simulink model "Tire_Force_Observer_Test"  (R2018b)
settings: Solver=VariableStepAuto  StartTime=0.0  StopTime=10  RelTol=1e-3  EnableMultiTasking=on
undefined symbols (not defined in the file or in its folder): A_s, B_s, C_s, Jw, K_s, r, sigbuilder_block, tyre_radius
libraries: simulink x1
settings Model: PauseTimes=1  Creator=univ4123  LastModifiedBy=univ4123
settings OptimizationCC: LifeSpan=inf
settings DebuggingCC: SFUnexpectedBacktrackingDiag=warning  SFNoUnconditionalDefaultTransitionDiag=warning
settings SFSimCC: SimUseLocalCustomCode=off
settings RTWCC: RTWUseLocalCustomCode=off
settings CodeAppCC: StateflowObjectComments=on
settings GRTTargetCC: TargetLangStandard=C89/C90 (ANSI)  GeneratePreprocessorConditionals=Disable all
settings ConfigComp: CovMetricSettings=dw  CovHtmlReporting=on  CovSaveCumulativeToWorkspaceVar=on  CovSaveSingleToWorkspaceVar=on  CovExternalEMLEnable=off

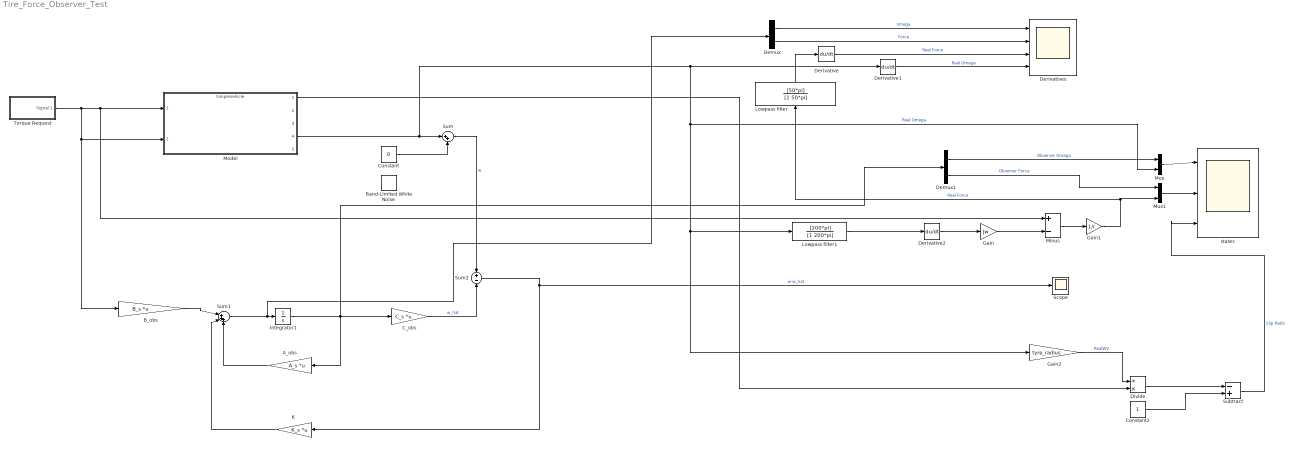
== system Tire_Force_Observer_Test ==
  A_obs : Gain  Gain=A_s  Multiplication=Matrix(K*u) (u vector)
  B_obs : Gain  Gain=B_s  Multiplication=Matrix(K*u) (u vector)
  Band-Limited White Noise : simulink/Sources/Band-Limited White Noise  Cov=[0.00001]  Ts=0.1  seed=[23341]
  C_obs : Gain  Gain=C_s  Multiplication=Matrix(K*u) (u vector)
  Constant : Constant  Value=0
  Constant2 : Constant
  Demux : Demux  Outputs=2
  Demux1 : Demux  Outputs=2
  Derivative : Derivative
  Derivative1 : Derivative
  Derivative2 : Derivative
  "Derivatives " : Scope  NumInputPorts=4
  Divide : Product  Inputs=/*
  Gain : Gain  Gain=Jw
  Gain1 : Gain  Gain=1/r
  Gain2 : Gain  Gain=tyre_radius
  Integrator1 : Integrator
  K : Gain  Gain=K_s  Multiplication=Matrix(K*u)
  Lowpass filter : TransferFcn  Numerator=[50*pi]  Denominator=[1 50*pi]
  Lowpass filter1 : TransferFcn  Numerator=[200*pi]  Denominator=[1 200*pi]
  Minus : Sum  Inputs=+-
  Model : ModelReference  ModelNameDialog=SimpleVehicle.slx  SimulationMode=Normal  ModelReferenceVersion=1.9
  Mux : Mux  Inputs=2
  Mux1 : Mux  Inputs=2
  Scope : Scope
  Subtract : Sum  Inputs=-+
  Sum : Sum  Inputs=|++
  Sum1 : Sum  Inputs=|+++
  Sum2 : Sum  Inputs=+|-
  Torque Request : Subsystem  Tag=STV Subsys  LoadFcn=sigbuilder_block('load');  StartFcn=sigbuilder_block('start');  StopFcn=sigbuilder_block('stop');  ClipboardFcn=sigbuilder_block('clipboard');  mask(Sigbuilder block){tuvar=[0:10]}
      mask help: Simulink:masks:SigbuilderBlock_MD
      mask init:
      | if ~strcmp(get_param(bdroot(gcbh),'SimulationStatus'),'stopped') tuvar = sigbuilder_block('maskInit'); end
      settings: CopyFcn=sigbuilder_block('copy');  DeleteFcn=sigbuilder_block('delete');  ModelCloseFcn=sigbuilder_block('modelClose');  PreSaveFcn=sigbuilder_block('preSave');  PauseFcn=sigbuilder_block('pause');  ContinueFcn=sigbuilder_block('continue');  NameChangeFcn=sigbuilder_block('namechange');  OpenFcn=sigbuilder_block('open',[437.6 153.75 550.4 359.25 ]);  CloseFcn=sigbuilder_block('close');
      mask Display: plot(0, 0, 100, 100,[2, 2, 32, 32, 2], [68, 8, 8, 68, 68],[32, 2], [38, 38], [32, 19, 2],[53, 60, 44], [32, 17, 17, 2],[16, 16, 31, 31]);txt = getActiveGroup(gcbh);text(2, 100, txt,'verticalAlignment', 'top');
  states : Scope  NumInputPorts=3
  wires:
  Sum1/1 -> Demux/1, Integrator1/1
  Demux1/1 -> Mux/1  "Observer Omega"
  Model/4 -> Gain2/1, Lowpass filter1/1, Mux/2, Derivative1/1, Sum/1  "Real Omega"
  Derivative/1 -> "Derivatives "/3  "Real Force"
  Sum/1 -> Sum2/1  "w"
  Integrator1/1 -> Demux1/1, A_obs/1, C_obs/1
  Constant/1 -> Sum/2
  B_obs/1 -> Sum1/1
  Demux1/2 -> Mux1/1  "Observer Force"
  Demux/2 -> "Derivatives "/2  "Force"
  A_obs/1 -> Sum1/3
  Demux/1 -> "Derivatives "/1  "omega"
  Torque Request/1(Signal 1) -> Model/1, Minus/1, Model/2, B_obs/1
  K/1 -> Sum1/2
  C_obs/1 -> Sum2/2  "w_hat"
  Sum2/1 -> Scope/1, K/1  "w-w_hat"
  Derivative1/1 -> "Derivatives "/4  "Real Omega"
  Derivative2/1 -> Gain/1
  Gain/1 -> Minus/2
  Minus/1 -> Gain1/1
  Gain1/1 -> Lowpass filter/1, Mux1/2  "Real Force"
  Gain2/1 -> Divide/1  "RealWV"
  Divide/1 -> Subtract/1
  Subtract/1 -> states/3  "Slip Ratio"
  Model/1 -> Divide/2
  Constant2/1 -> Subtract/2
  Mux/1 -> states/1
  Mux1/1 -> states/2
  Lowpass filter/1 -> Derivative/1
  Lowpass filter1/1 -> Derivative2/1

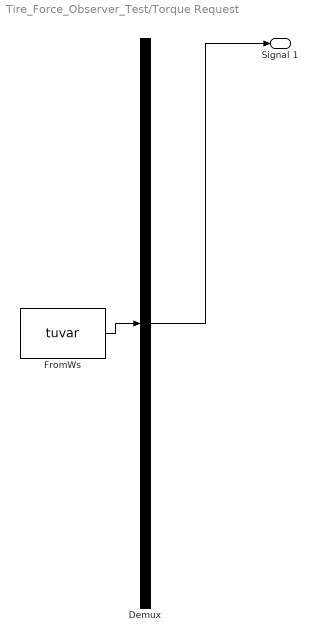
== system Tire_Force_Observer_Test/Torque Request ==
  Demux : Demux  Tag=STV Demux  Outputs=1
  FromWs : FromWorkspace  Tag=STV FromWs  VariableName=tuvar  SampleTime=0
      SigBuilderData=|
      | common.afterFinalStr = 'Extrapolate'
      | common.sampleTime = 0
      | dataSet.timeRange = [0 10]
      | dataSet.name = 'Group 1'
      | sbobj.Groups.Name = 'Group 1'
      | sbobj.Groups.Signals.Name = 'Signal 1'
      | sbobj.Groups.Signals.XData = [0 1 1.5 5.5 6 10]
      | sbobj.Groups.Signals.YData = [0 0 120 200 0 0]
  Signal 1 : Outport  Tag=STV Outport
  wires:
  Demux/1 -> Signal 1/1
  FromWs/1 -> Demux/1
